simulink model "osuWorkshop"  (R2023b)
settings: Solver=FixedStepDiscrete  StartTime=0.0  StopTime=inf  FixedStep=Ts  RelTol=1e-3
values from neighbouring files (symbols this model uses):
  loadCellScale = loadCellMaxN/(el3751Scale*loadCellCal)    [init.m]
  Ts = 1/1000    (= 0.001)    [init.m]
undefined symbols (not defined in the file or in its folder): acknError, actuatorStatusStruct, ctrlStruct, current_A, eCatDcErr, eCatDcInit, eCatErr, eCatLastErr, eCatMnClkDiff, eCatNsClkDiff, eCatState, eCatStatusStruct, force_N, home, homed, opEnabled, position_m, specialMode, state, switchOn, velocity_m_s
libraries: slrealtimeethercatlib x11, slrealtimeloglib x2, slrealtimeutilitieslib x1
settings Model: Creator=Johannes  LastModifiedBy=jspin
settings SolverCC: ConcurrentTasks=on  PositivePriorityOrder=on
settings OptimizationCC: BlockReduction=off  OptimizeBlockIOStorage=off  ReuseModelBlockBuffer=off
settings DebuggingCC: TasksWithSamePriorityMsg=none
settings HardwareCC: ProdBitPerLong=64  ProdLongLongMode=on  ProdHWDeviceType=Intel->x86-64 (Linux 64)
settings RTWCC: Description=Simulink Real-Time  SystemTargetFile=slrealtime.tlc  TemplateMakefile=slrealtime_default_tmf  RTWVerbose=off  Toolchain=Simulink Real-Time Toolchain  BuildConfiguration=Faster Runs  CodeExecutionProfiling=on  TargetLang=C++

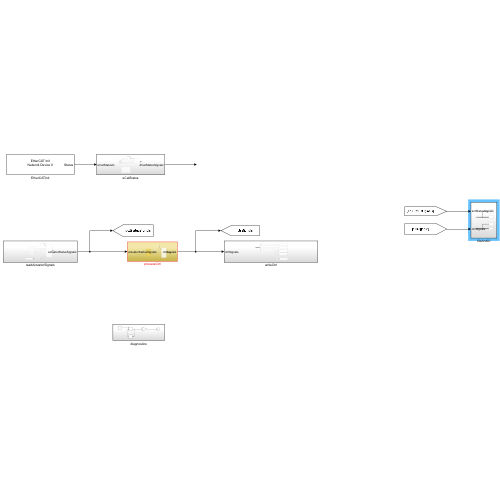
[thumbnail: Simulink's stored preview of the top-level diagram]
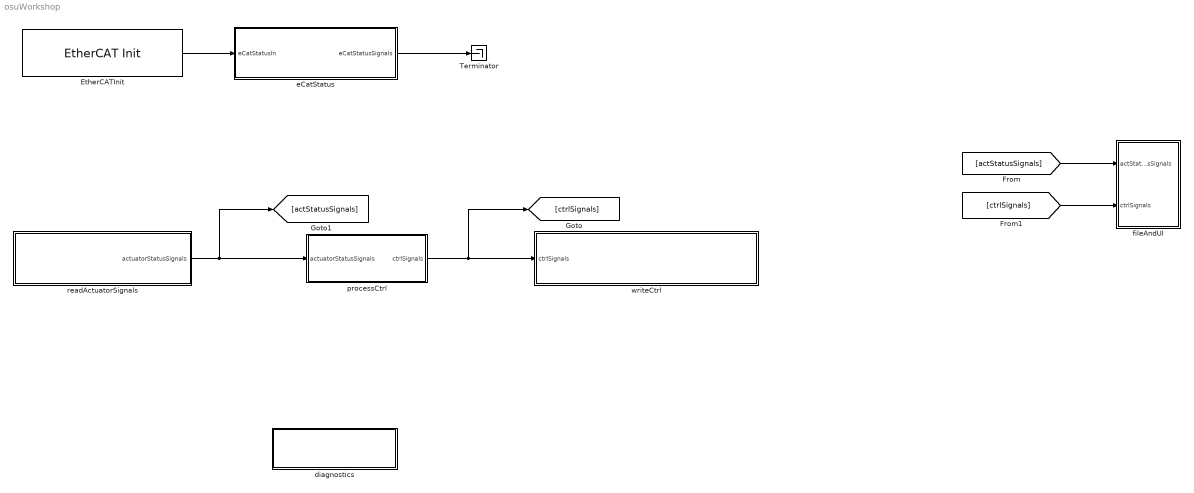
== system osuWorkshop ==
  EtherCATInit : slrealtimeethercatlib/EtherCAT Init  Priority=0  config_file=D:\src\egi\osu-workshop\ethercat\OSUWorkshopENI.xml  device_id=0  portnum=1  initstate=2  dctuning=0  enaDebug=0  logFile='c:\dbglog.txt'  sample_time=0.001000  DCMode=0
  Terminator : Terminator
  diagnostics : Subsystem
  eCatStatus : Subsystem
  fileAndUI : Subsystem
  processCtrl : Subsystem
  readActuatorSignals : Subsystem
  writeCtrl : Subsystem
  wires:
  EtherCATInit/1 -> eCatStatus/1(eCatStatusIn)
  readActuatorSignals/1(actuatorStatusSignals) -> [actStatusSignals], processCtrl/1(actuatorStatusSignals)
  processCtrl/1(ctrlSignals) -> [ctrlSignals], writeCtrl/1(ctrlSignals)
  eCatStatus/1(eCatStatusSignals) -> Terminator/1
  [actStatusSignals] -> fileAndUI/1(actStatusSignals)
  [ctrlSignals] -> fileAndUI/2(ctrlSignals)

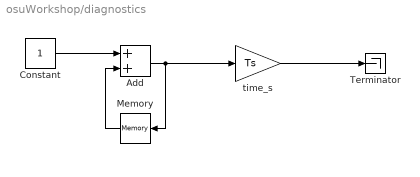
== system osuWorkshop/diagnostics ==
  Add : Sum
  Constant : Constant
  Memory : Memory
  Terminator : Terminator
  time_s : Gain  Gain=Ts
  wires:
  Add/1 -> time_s/1, Memory/1
  Memory/1 -> Add/2
  Constant/1 -> Add/1
  time_s/1 -> Terminator/1

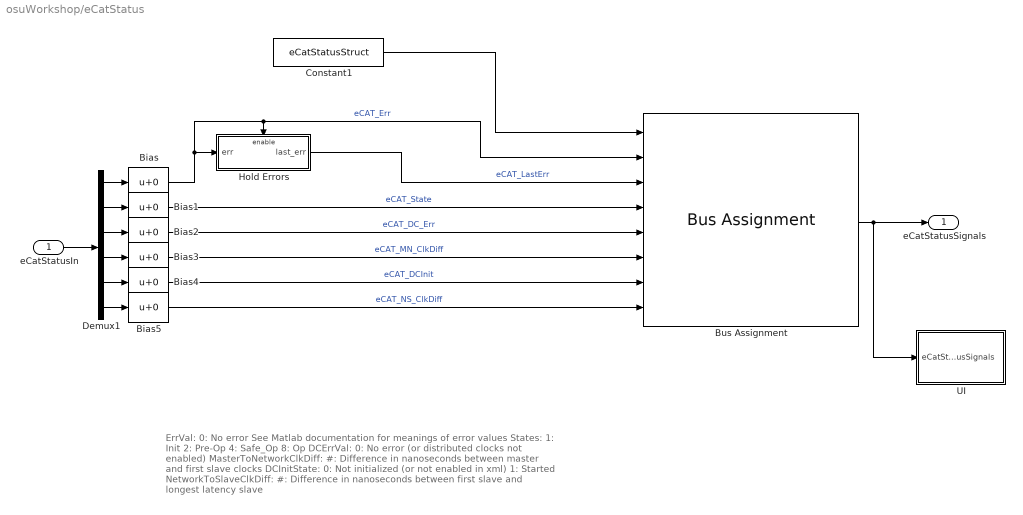
== system osuWorkshop/eCatStatus ==
  note: ErrVal:
      | 	0: No error
      | 	See Matlab documentation for meanings of error values
      | States:
      | 	1: Init
      | 	2: Pre-Op
      | 	4: Safe_Op
      | 	8: Op
      | DCErrVal:
      | 	0: No error (or distributed clocks not enabled)
      | MasterToNetworkClkDiff:
      | 	#: Difference in nanoseconds between master and first slave clocks
      | DCInitState:
      | 	0: Not initialized (or not enabled in xml)
      | 	1: Started
      | NetworkToSlaveClkDiff:
      | 	#: Difference in nanoseconds between first slave and longest latency slave
  eCatStatusIn : Inport
  Bias{,1..5} (6 alike) : Bias  SaturateOnIntegerOverflow=off
  Bus Assignment : BusAssignment  AssignedSignals=eCatErr,eCatLastErr,eCatState,eCatDcErr,eCatMnClkDiff,eCatDcInit,eCatNsClkDiff
  Constant1 : Constant  Value=eCatStatusStruct  OutDataTypeStr=Bus: eCatStatusBus
  Demux1 : Demux  Outputs=6
  Hold Errors : Subsystem  TreatAsAtomicUnit=on
  UI : Subsystem
  eCatStatusSignals : Outport  OutDataTypeStr=Bus: eCatStatusBus
  wires:
  Bias1/1 -> Bus Assignment/4  "eCAT_State"
  eCatStatusIn/1 -> Demux1/1
  Hold Errors/1(last_err) -> Bus Assignment/3  "eCAT_LastErr"
  Bias5/1 -> Bus Assignment/8  "eCAT_NS_ClkDiff"
  Bias/1 -> Bus Assignment/2, Hold Errors/Enable, Hold Errors/1(err)  "eCAT_Err"
  Demux1/3 -> Bias2/1
  Bus Assignment/1 -> UI/1(eCatStatusSignals), eCatStatusSignals/1
  Bias3/1 -> Bus Assignment/6  "eCAT_MN_ClkDiff"
  Demux1/6 -> Bias5/1
  Demux1/2 -> Bias1/1
  Bias2/1 -> Bus Assignment/5  "eCAT_DC_Err"
  Bias4/1 -> Bus Assignment/7  "eCAT_DCInit"
  Demux1/1 -> Bias/1
  Demux1/5 -> Bias4/1
  Demux1/4 -> Bias3/1
  Constant1/1 -> Bus Assignment/1

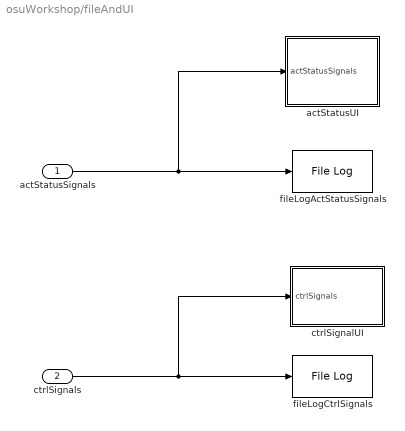
== system osuWorkshop/fileAndUI ==
  actStatusSignals : Inport  OutDataTypeStr=Bus: actuatorStatusBus
  ctrlSignals : Inport  Port=2  OutDataTypeStr=Bus: ctrlBus
  actStatusUI : Subsystem
  ctrlSignalUI : Subsystem
  fileLogActStatusSignals : slrealtimeloglib/File Log  decimation=fileDecimation  inputProcessing=Elements as channels (sample based)
  fileLogCtrlSignals : slrealtimeloglib/File Log  decimation=fileDecimation  inputProcessing=Elements as channels (sample based)
  wires:
  actStatusSignals/1 -> actStatusUI/1(actStatusSignals), fileLogActStatusSignals/1
  ctrlSignals/1 -> ctrlSignalUI/1(ctrlSignals), fileLogCtrlSignals/1

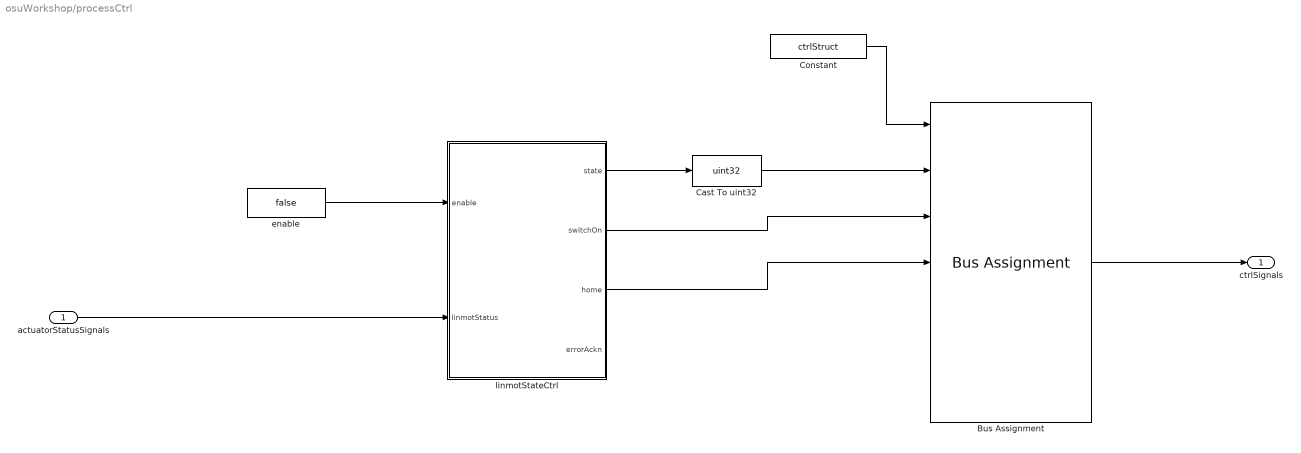
== system osuWorkshop/processCtrl ==
  actuatorStatusSignals : Inport
  Bus Assignment : BusAssignment  AssignedSignals=state,switchOn,home,specialMode,acknError,current_A
  Cast To uint32 : DataTypeConversion  OutDataTypeStr=uint32  SaturateOnIntegerOverflow=off  RndMeth=Floor
  Constant : Constant  Value=ctrlStruct  OutDataTypeStr=Bus: ctrlBus
  enable : Constant  Value=false  OutDataTypeStr=boolean
  linmotStateCtrl : Stateflow chart  TreatAsAtomicUnit=on
  ctrlSignals : Outport  OutDataTypeStr=Bus: ctrlBus
  wires:
  Bus Assignment/1 -> ctrlSignals/1
  Constant/1 -> Bus Assignment/1
  enable/1 -> linmotStateCtrl/1(enable)
  Cast To uint32/1 -> Bus Assignment/2
  linmotStateCtrl/1(state) -> Cast To uint32/1
  linmotStateCtrl/2(switchOn) -> Bus Assignment/3
  linmotStateCtrl/3(home) -> Bus Assignment/4
  actuatorStatusSignals/1 -> linmotStateCtrl/2(linmotStatus)

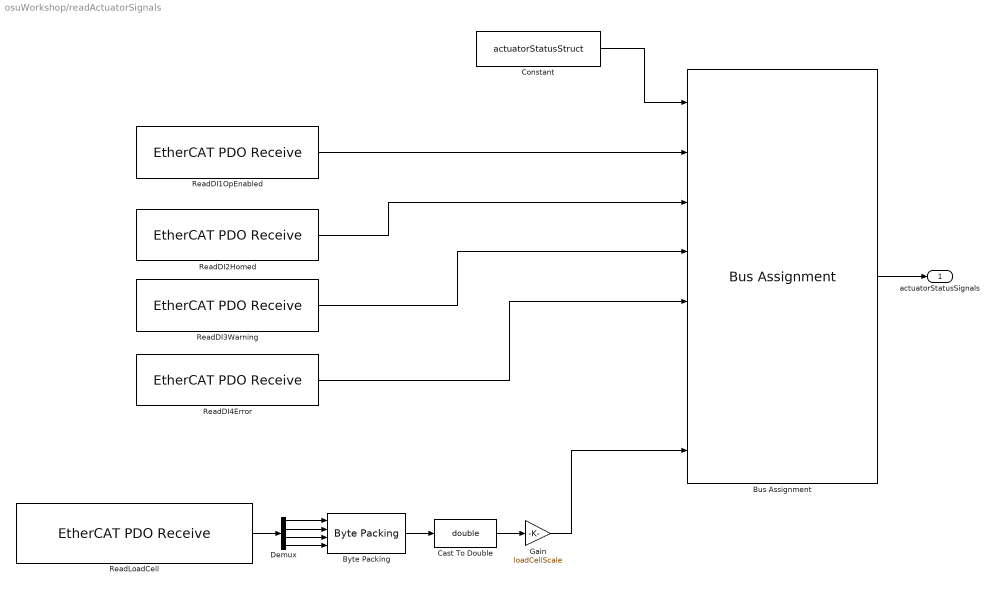
== system osuWorkshop/readActuatorSignals ==
  Bus Assignment : BusAssignment  AssignedSignals=opEnabled,homed,warning,error,position_m,velocity_m_s,force_N
  Byte Packing : slrealtimeutilitieslib/Byte Packing  MaskPackedDataType=int32  MaskUnpackedDataTypes={'uint8','uint8','uint8','uint8'}  MaskAlignment=1
  Cast To Double : DataTypeConversion  OutDataTypeStr=double  SaturateOnIntegerOverflow=off  RndMeth=Floor
  Constant : Constant  Value=actuatorStatusStruct  OutDataTypeStr=Bus: actuatorStatusBus
  Demux : Demux
  Gain : Gain  Gain=loadCellScale
  ReadDI1OpEnabled : slrealtimeethercatlib/EtherCAT PDO Receive  Priority=2  sig_name=Main_EL1004_01.Channel 1.Input  sig_offset=704  sig_type=boolean  type_size=1  sig_dim=1  device_id=0  sample_time=0.001000
  ReadDI2Homed : slrealtimeethercatlib/EtherCAT PDO Receive  Priority=2  sig_name=Main_EL1004_01.Channel 2.Input  sig_offset=705  sig_type=boolean  type_size=1  sig_dim=1  device_id=0  sample_time=0.001000
  ReadDI3Warning : slrealtimeethercatlib/EtherCAT PDO Receive  Priority=2  sig_name=Main_EL1004_01.Channel 3.Input  sig_offset=706  sig_type=boolean  type_size=1  sig_dim=1  device_id=0  sample_time=0.001000
  ReadDI4Error : slrealtimeethercatlib/EtherCAT PDO Receive  Priority=2  sig_name=Main_EL1004_01.Channel 4.Input  sig_offset=707  sig_type=boolean  type_size=1  sig_dim=1  device_id=0  sample_time=0.001000
  ReadLoadCell : slrealtimeethercatlib/EtherCAT PDO Receive  Priority=2  sig_name=Main_EL3751_01.PAI Samples 1.Samples  sig_offset=608  sig_type=uint8  type_size=8  sig_dim=4  device_id=0  sample_time=0.001000
  actuatorStatusSignals : Outport  OutDataTypeStr=Bus: actuatorStatusBus
  wires:
  Gain/1 -> Bus Assignment/8
  Cast To Double/1 -> Gain/1
  Demux/2 -> Byte Packing/2
  Demux/4 -> Byte Packing/4
  Demux/3 -> Byte Packing/3
  Demux/1 -> Byte Packing/1
  Byte Packing/1 -> Cast To Double/1
  ReadLoadCell/1 -> Demux/1
  Constant/1 -> Bus Assignment/1
  ReadDI1OpEnabled/1 -> Bus Assignment/2
  ReadDI2Homed/1 -> Bus Assignment/3
  ReadDI3Warning/1 -> Bus Assignment/4
  ReadDI4Error/1 -> Bus Assignment/5
  Bus Assignment/1 -> actuatorStatusSignals/1

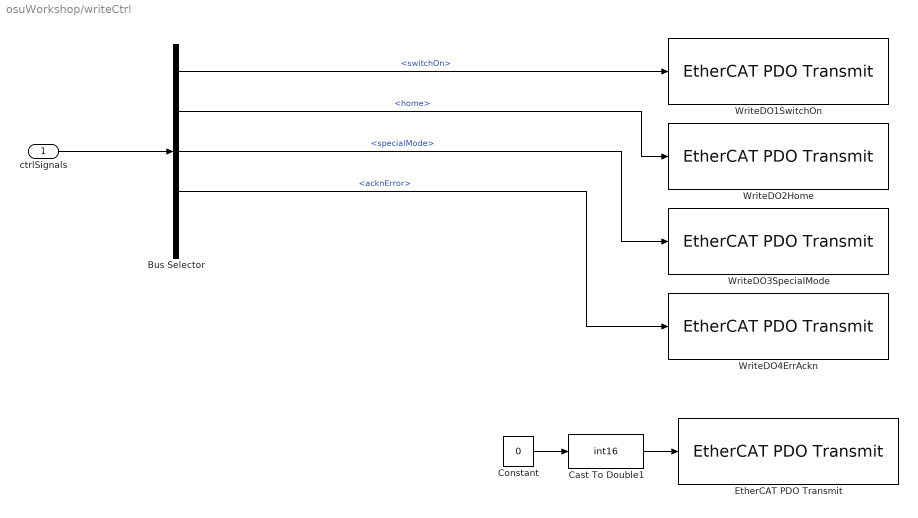
== system osuWorkshop/writeCtrl ==
  ctrlSignals : Inport  OutDataTypeStr=Bus: ctrlBus
  Bus Selector : BusSelector  OutputSignals=switchOn,home,specialMode,acknError,current_A
  Cast To Double1 : DataTypeConversion  OutDataTypeStr=int16  SaturateOnIntegerOverflow=off  RndMeth=Floor
  Constant : Constant  Value=0
  EtherCAT PDO Transmit : slrealtimeethercatlib/EtherCAT PDO Transmit  Priority=3  sig_name=Main_EL4132_01.Channel 1.Output  sig_offset=440  sig_type=int16  type_size=16  sig_dim=1  device_id=0  sample_time=0.001000
  WriteDO1SwitchOn : slrealtimeethercatlib/EtherCAT PDO Transmit  Priority=3  sig_name=Main_EL2004_01.Channel 1.Output  sig_offset=472  sig_type=boolean  type_size=1  sig_dim=1  device_id=0  sample_time=0.001000
  WriteDO2Home : slrealtimeethercatlib/EtherCAT PDO Transmit  Priority=3  sig_name=Main_EL2004_01.Channel 2.Output  sig_offset=473  sig_type=boolean  type_size=1  sig_dim=1  device_id=0  sample_time=0.001000
  WriteDO3SpecialMode : slrealtimeethercatlib/EtherCAT PDO Transmit  Priority=3  sig_name=Main_EL2004_01.Channel 3.Output  sig_offset=474  sig_type=boolean  type_size=1  sig_dim=1  device_id=0  sample_time=0.001000
  WriteDO4ErrAckn : slrealtimeethercatlib/EtherCAT PDO Transmit  Priority=3  sig_name=Main_EL2004_01.Channel 4.Output  sig_offset=475  sig_type=boolean  type_size=1  sig_dim=1  device_id=0  sample_time=0.001000
  wires:
  Constant/1 -> Cast To Double1/1
  Cast To Double1/1 -> EtherCAT PDO Transmit/1
  ctrlSignals/1 -> Bus Selector/1
  Bus Selector/1 -> WriteDO1SwitchOn/1  "<switchOn>"
  Bus Selector/2 -> WriteDO2Home/1  "<home>"
  Bus Selector/3 -> WriteDO3SpecialMode/1  "<specialMode>"
  Bus Selector/4 -> WriteDO4ErrAckn/1  "<acknError>"

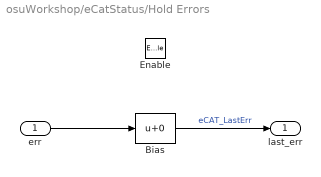
== system osuWorkshop/eCatStatus/Hold Errors ==
  err : Inport
  Enable : EnablePort
  Bias : Bias  SaturateOnIntegerOverflow=off
  last_err : Outport
  wires:
  err/1 -> Bias/1
  Bias/1 -> last_err/1  "eCAT_LastErr"

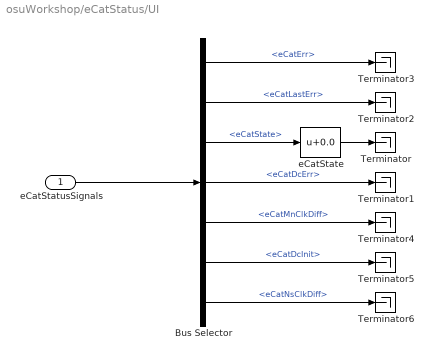
== system osuWorkshop/eCatStatus/UI ==
  eCatStatusSignals : Inport  OutDataTypeStr=Bus: eCatStatusBus
  Bus Selector : BusSelector  OutputSignals=eCatErr,eCatLastErr,eCatState,eCatDcErr,eCatMnClkDiff,eCatDcInit,eCatNsClkDiff
  Terminator{,1..6} (7 alike) : Terminator
  eCatState : Bias  Bias=0.0  SaturateOnIntegerOverflow=off
  wires:
  eCatStatusSignals/1 -> Bus Selector/1
  Bus Selector/3 -> eCatState/1  "<eCatState>"
  eCatState/1 -> Terminator/1
  Bus Selector/4 -> Terminator1/1  "<eCatDcErr>"
  Bus Selector/2 -> Terminator2/1  "<eCatLastErr>"
  Bus Selector/1 -> Terminator3/1  "<eCatErr>"
  Bus Selector/5 -> Terminator4/1  "<eCatMnClkDiff>"
  Bus Selector/6 -> Terminator5/1  "<eCatDcInit>"
  Bus Selector/7 -> Terminator6/1  "<eCatNsClkDiff>"

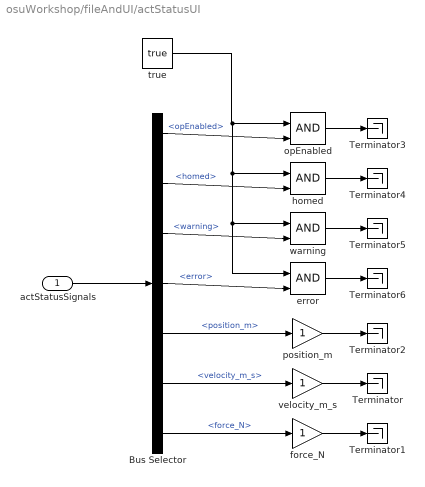
== system osuWorkshop/fileAndUI/actStatusUI ==
  actStatusSignals : Inport  OutDataTypeStr=Bus: actuatorStatusBus
  Bus Selector : BusSelector  OutputSignals=opEnabled,homed,warning,error,position_m,velocity_m_s,force_N
  Terminator{,1..6} (7 alike) : Terminator
  error : Logic  IconShape=distinctive  AllPortsSameDT=off  OutDataTypeStr=boolean
  force_N : Gain
  homed : Logic  IconShape=distinctive  AllPortsSameDT=off  OutDataTypeStr=boolean
  opEnabled : Logic  IconShape=distinctive  AllPortsSameDT=off  OutDataTypeStr=boolean
  position_m : Gain
  true : Constant  Value=true  OutDataTypeStr=boolean
  velocity_m_s : Gain
  warning : Logic  IconShape=distinctive  AllPortsSameDT=off  OutDataTypeStr=boolean
  wires:
  actStatusSignals/1 -> Bus Selector/1
  Bus Selector/7 -> force_N/1  "<force_N>"
  Bus Selector/6 -> velocity_m_s/1  "<velocity_m_s>"
  velocity_m_s/1 -> Terminator/1
  force_N/1 -> Terminator1/1
  Bus Selector/5 -> position_m/1  "<position_m>"
  position_m/1 -> Terminator2/1
  Bus Selector/1 -> opEnabled/2  "<opEnabled>"
  Bus Selector/2 -> homed/2  "<homed>"
  Bus Selector/3 -> warning/2  "<warning>"
  Bus Selector/4 -> error/2  "<error>"
  opEnabled/1 -> Terminator3/1
  homed/1 -> Terminator4/1
  warning/1 -> Terminator5/1
  error/1 -> Terminator6/1
  true/1 -> error/1, warning/1, homed/1, opEnabled/1

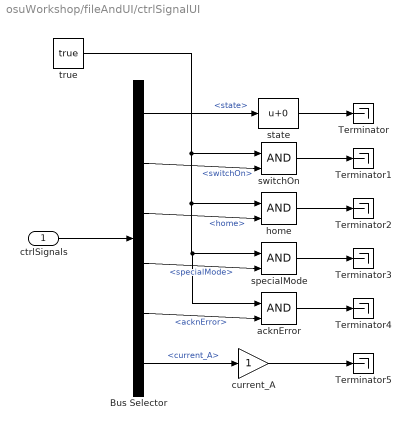
== system osuWorkshop/fileAndUI/ctrlSignalUI ==
  ctrlSignals : Inport  OutDataTypeStr=Bus: ctrlBus
  Bus Selector : BusSelector  OutputSignals=state,switchOn,home,specialMode,acknError,current_A
  Terminator{,1..5} (6 alike) : Terminator
  acknError : Logic  IconShape=distinctive  AllPortsSameDT=off  OutDataTypeStr=boolean
  current_A : Gain
  home : Logic  IconShape=distinctive  AllPortsSameDT=off  OutDataTypeStr=boolean
  specialMode : Logic  IconShape=distinctive  AllPortsSameDT=off  OutDataTypeStr=boolean
  state : Bias  SaturateOnIntegerOverflow=off
  switchOn : Logic  IconShape=distinctive  AllPortsSameDT=off  OutDataTypeStr=boolean
  true : Constant  Value=true  OutDataTypeStr=boolean
  wires:
  ctrlSignals/1 -> Bus Selector/1
  Bus Selector/6 -> current_A/1  "<current_A>"
  Bus Selector/2 -> switchOn/2  "<switchOn>"
  Bus Selector/3 -> home/2  "<home>"
  true/1 -> acknError/1, specialMode/1, home/1, switchOn/1
  Bus Selector/4 -> specialMode/2  "<specialMode>"
  Bus Selector/5 -> acknError/2  "<acknError>"
  Bus Selector/1 -> state/1  "<state>"
  state/1 -> Terminator/1
  switchOn/1 -> Terminator1/1
  home/1 -> Terminator2/1
  specialMode/1 -> Terminator3/1
  acknError/1 -> Terminator4/1
  current_A/1 -> Terminator5/1

== stateflow chart osuWorkshop/processCtrl/linmotStateCtrl ==
  state init
    entry:
    state = linmotStateEnum.init;
    switchOn = false;
    home = false;
    errorAckn = false;
  state readyToEnable
    entry:
    state = linmotStateEnum.readyToEnable;
    switchOn = false;
    home = false;
    errorAckn = false;
  state switchingOn
    entry:
    state = linmotStateEnum.switchingOn;
    switchOn = true;
    home = false;
    errorAckn = false;
  state homing
    entry:
    state = linmotStateEnum.homing;
    switchOn = true;
    home = true;
    errorAckn = false;
  state enabled
    entry:
    state = linmotStateEnum.enabled;
    switchOn = true;
    home = false;
    errorAckn = false;
  state error
    entry:
    switchOn = false;
    home = false;
    errorAckn = false;
  (default) -> init
  (junction 46) -> init
  (junction 37) -> (junction 46)
  init -> (junction 4) [order 1] : [linmotStatus.error]
  (junction 4) -> (junction 9)
  init -> readyToEnable [order 2] : [after(2,'sec')] % enter readyToEnable if no error
  readyToEnable -> (junction 9) [order 1] : [linmotStatus.error]
  (junction 9) -> (junction 20)
  readyToEnable -> switchingOn [order 2] : [enable]
  switchingOn -> (junction 20) [order 2] : [linmotStatus.error]
  switchingOn -> (junction 37) [order 3] : [~enable]
  (junction 20) -> (junction 21)
  (junction 40) -> (junction 37)
  switchingOn -> homing [order 1] : [linmotStatus.opEnabled]
  homing -> (junction 40) [order 3] : [~enable]
  homing -> (junction 21) [order 2] : [linmotStatus.error]
  (junction 42) -> (junction 40)
  (junction 21) -> (junction 22)
  homing -> enabled [order 1] : [after(2,'sec') && linmotStatus.homed] % timeout to ensure home is not latched
  enabled -> (junction 42) [order 2] : [~enable]
  (junction 22) -> error
  enabled -> (junction 22) [order 1] : [linmotStatus.error]
  data: state output Enum: linmotStateEnum; switchOn output boolean; home output boolean; enable input boolean; errorAckn output boolean; linmotStatus input Bus: actuatorStatusBus
